simulink model "mdl_pm_foc_allpu_alternative"  (R2024a)
settings: Solver=FixedStepAuto  StartTime=0.0  StopTime=1  FixedStep=1e-5  RelTol=1e-3
undefined symbols (not defined in the file): param, sigbuilder_block
libraries: spsControlledVoltageSourceLib x3, spsPermanentMagnetSynchronousMachineLib x1, spsGroundLib x1, sps_lib x1
settings Model: Creator=jack  LastModifiedBy=steve
settings SolverCC: ZeroCrossControl=DisableAll  ZeroCrossAlgorithm=Adaptive
settings OptimizationCC: ReuseModelBlockBuffer=off
settings DebuggingCC: MaskedZcDiagnostic=none  IgnoredZcDiagnostic=none
settings RTWCC: GPUComputeCapability=3.5

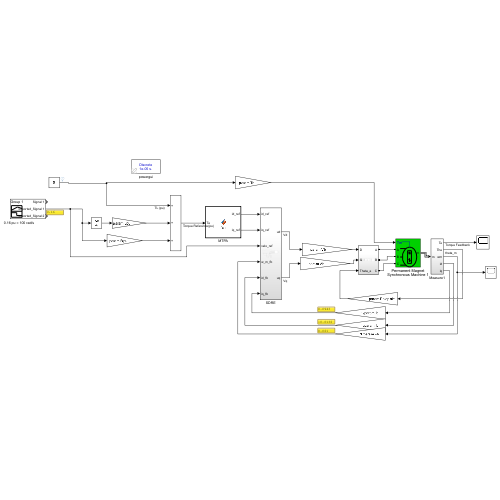
[thumbnail: Simulink's stored preview of the top-level diagram]
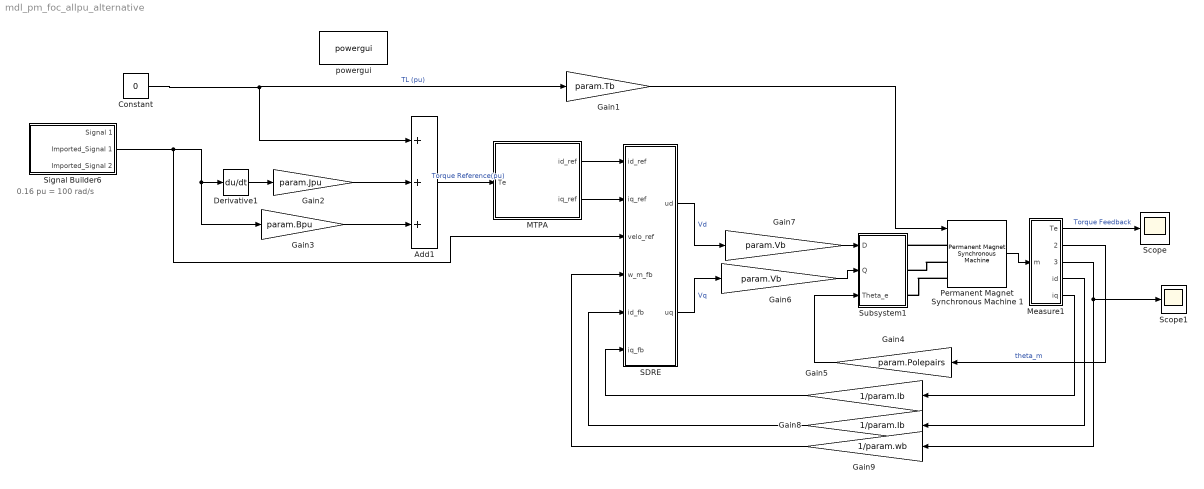
== system mdl_pm_foc_allpu_alternative ==
  note: 0.16 pu = 100 rad/s
  Add1 : Sum  Inputs=+++
  Constant : Constant  Value=0
  Derivative1 : Derivative
  Gain1 : Gain  Gain=param.Tb
  Gain2 : Gain  Gain=param.Jpu
  Gain3 : Gain  Gain=param.Bpu
  Gain4 : Gain  Gain=param.Polepairs
  Gain5 : Gain  Gain=1/param.Ib
  Gain6 : Gain  Gain=param.Vb
  Gain7 : Gain  Gain=param.Vb
  Gain8 : Gain  Gain=1/param.Ib
  Gain9 : Gain  Gain=1/param.wb
  MTPA : MATLAB Function  TreatAsAtomicUnit=on
  Measure1 : Subsystem
  Permanent Magnet Synchronous Machine 1 : spsPermanentMagnetSynchronousMachineLib/Permanent Magnet Synchronous Machine  NbPhases=3  FluxDistribution=Sinusoidal  RotorType=Salient-pole  MechanicalLoad=Torque Tm  PresetModel=No  ShowDetailedParameters=on  MeasurementBus=off  Resistance=param.Rs  Inductance=8.5e-3  dqInductances=[param.Ld param.Lq]  La=5.7e-3  MachineConstant=Flux linkage established by magnets (V.s)  Flux=param.Lamda_f  VoltageCst=164.1942  TorqueCst=1.3579  Flat=120  Mechanical=[param.J param.B param.Polepairs]  PolePairs=4  InitialConditions=[0,0, 0,0]  InitialConditions5ph=[0 0 0 0 0 0]  RefAngle=Aligned with phase A axis (original Park)  IterativeDiscreteModel=Trapezoidal non iterative  TsBlock=param.timestep  TsPowergui=0
  SDRE : Subsystem
  Scope : Scope
  Scope1 : Scope
  Signal Builder6 : Subsystem  Tag=STV Subsys  LoadFcn=sigbuilder_block('load');  StartFcn=sigbuilder_block('start');  StopFcn=sigbuilder_block('stop');  ClipboardFcn=sigbuilder_block('clipboard');  mask(Sigbuilder block){tuvar=[0:10]}
      mask help: Simulink:masks:SigbuilderBlock_MD
      mask init:
      | if ~strcmp(get_param(bdroot(gcbh),'SimulationStatus'),'stopped') tuvar = sigbuilder_block('maskInit'); end
      settings: CopyFcn=sigbuilder_block('copy');  DeleteFcn=sigbuilder_block('delete');  ModelCloseFcn=sigbuilder_block('modelClose');  PreSaveFcn=sigbuilder_block('preSave');  PauseFcn=sigbuilder_block('pause');  ContinueFcn=sigbuilder_block('continue');  NameChangeFcn=sigbuilder_block('namechange');  OpenFcn=sigbuilder_block('open',[6 0 1428 711.75 ]);  CloseFcn=sigbuilder_block('close');
      mask Display: plot(0, 0, 100, 100,[2, 2, 32, 32, 2], [68, 8, 8, 68, 68],[32, 2], [38, 38], [32, 19, 2],[53, 60, 44], [32, 17, 17, 2],[16, 16, 31, 31]);txt = getActiveGroup(gcbh);text(2, 100, txt,'verticalAlignment', 'top');
  Subsystem1 : Subsystem
  powergui : sps_lib/powergui  Priority=1  SimulationMode=Discrete  SampleTime=1e-05  frequency=60  Iterations=50  frequencyindice=0  Pbase=100e6  ErrMax=1e-4  UnitsV=kV  UnitsW=MW  buscounter=0  FunctionMessages=off  echomessages=off  EnableUseOfTLC=off  CurrentSourceSwitches=off  DisableSnubberDevices=off  DisableRonSwitches=off  DisableVfSwitches=off  DisplayEquations=off  AutomaticDiscreteSolvers=off  SolverType=Tustin/Backward Euler (TBE)  Interpol=off  ExternalGateDelay=off  methode=off  Ts=100  x0status=blocks  SPID=on  SwTol=0  HookPort=off  NonlinearTolerance=1e-4  nMaxIteration=100  ContinueOnMaxIteration=off  RestoreLinks=warning  ResistiveCurrentMeasurement=off  Frange=[0:2:500]  Ylog=off  Xlog=on  ShowGrid=off  save=off  variable=ZData  structure=0  ZoomFFT=off  StartTime=0.0  cycles=1  DisplayStyle=1  fundamental=60  FreqAxis=off  MaxFrequency=1000  frequencyindicesteady=1  RmsSteady=1  display=off
  wires:
  Constant/1 -> Add1/1, Gain1/1  "TL (pu)"
  Gain3/1 -> Add1/3
  Add1/1 -> MTPA/1(Te)  "Torque Reference(pu)"
  Gain2/1 -> Add1/2
  Signal Builder6/2(Imported_Signal 1) -> Gain3/1, Derivative1/1, SDRE/3(velo_ref)
  MTPA/1(id_ref) -> SDRE/1(id_ref)
  Derivative1/1 -> Gain2/1
  MTPA/2(iq_ref) -> SDRE/2(iq_ref)
  SDRE/2(uq) -> Gain6/1  "Vq"
  SDRE/1(ud) -> Gain7/1  "Vd"
  Permanent Magnet Synchronous Machine 1/1 -> Measure1/1(m)
  Gain1/1 -> Permanent Magnet Synchronous Machine 1/1
  Measure1/2(The) -> Gain4/1  "theta_m"
  Gain4/1 -> Subsystem1/3(Theta_e)
  Gain6/1 -> Subsystem1/2(Q)
  Gain7/1 -> Subsystem1/1(D)
  Measure1/5(iq) -> Gain5/1
  Measure1/4(id) -> Gain8/1
  Gain5/1 -> SDRE/6(iq_fb)
  Gain8/1 -> SDRE/5(id_fb)
  Gain9/1 -> SDRE/4(w_m_fb)
  Measure1/1(Te) -> Scope/1  "Torque Feedback"
  Measure1/3(wm) -> Scope1/1, Gain9/1
  connections:
  Permanent Magnet Synchronous Machine 1/LConn3 -- Subsystem1/RConn3
  Permanent Magnet Synchronous Machine 1/LConn2 -- Subsystem1/RConn2
  Permanent Magnet Synchronous Machine 1/LConn1 -- Subsystem1/RConn1

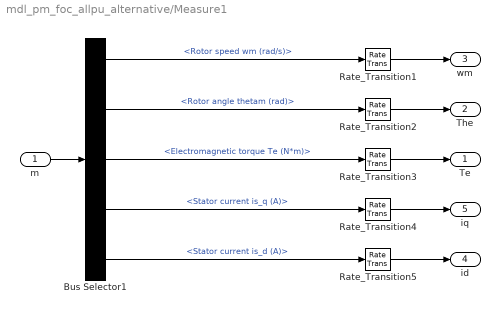
== system mdl_pm_foc_allpu_alternative/Measure1 ==
  m : Inport
  Bus Selector1 : BusSelector  OutputSignals=Rotor speed wm (rad/s),Rotor angle thetam (rad),Electromagnetic torque Te (N*m),Stator current is_q (A),Stator current is_d (A)
  Rate_Transition{1..5} (5 alike) : RateTransition  Integrity=off
  Te : Outport
  The : Outport  Port=2
  wm : Outport  Port=3
  id : Outport  Port=4
  iq : Outport  Port=5
  wires:
  Bus Selector1/1 -> Rate_Transition1/1  "<Rotor speed wm (rad/s)>"
  m/1 -> Bus Selector1/1
  Bus Selector1/3 -> Rate_Transition3/1  "<Electromagnetic torque Te (N*m)>"
  Bus Selector1/2 -> Rate_Transition2/1  "<Rotor angle thetam (rad)>"
  Rate_Transition1/1 -> wm/1
  Rate_Transition2/1 -> The/1
  Rate_Transition3/1 -> Te/1
  Bus Selector1/4 -> Rate_Transition4/1  "<Stator current is_q (A)>"
  Rate_Transition4/1 -> iq/1
  Bus Selector1/5 -> Rate_Transition5/1  "<Stator current is_d (A)>"
  Rate_Transition5/1 -> id/1

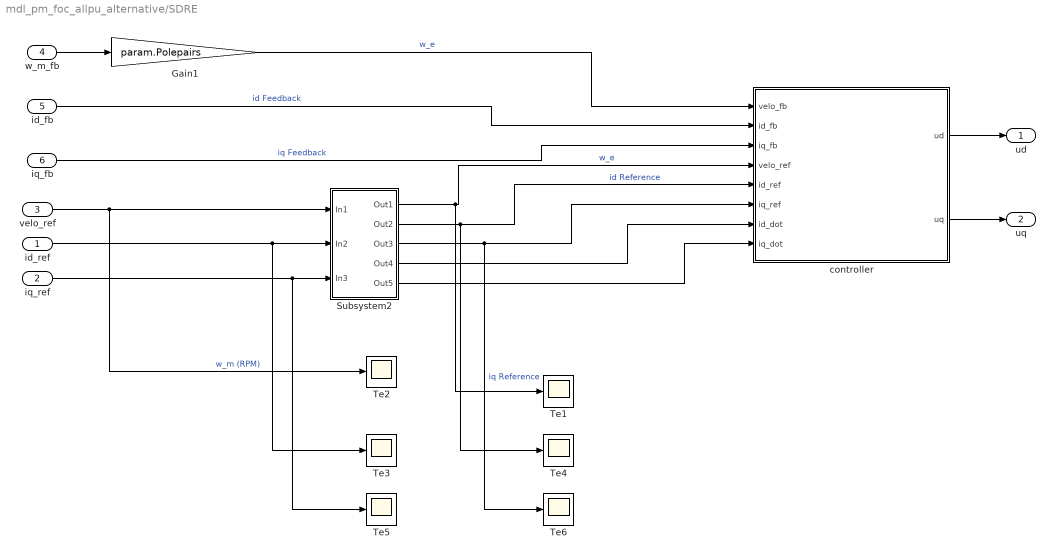
== system mdl_pm_foc_allpu_alternative/SDRE ==
  id_ref : Inport
  iq_ref : Inport  Port=2
  velo_ref : Inport  Port=3
  w_m_fb : Inport  Port=4
  id_fb : Inport  Port=5
  iq_fb : Inport  Port=6
  Gain1 : Gain  Gain=param.Polepairs
  Subsystem2 : Subsystem
  Te{1..6} (6 alike) : Scope
  controller : MATLAB Function  TreatAsAtomicUnit=on
  ud : Outport
  uq : Outport  Port=2
  wires:
  controller/2(uq) -> uq/1
  controller/1(ud) -> ud/1
  iq_ref/1 -> Te5/1, Subsystem2/3(In3)
  id_ref/1 -> Te3/1, Subsystem2/2(In2)
  velo_ref/1 -> Te2/1, Subsystem2/1(In1)  "w_m (RPM)"
  Subsystem2/5(Out5) -> controller/8(iq_dot)
  Subsystem2/4(Out4) -> controller/7(id_dot)
  Subsystem2/1(Out1) -> Te1/1, controller/4(velo_ref)  "w_e"
  Subsystem2/2(Out2) -> controller/5(id_ref), Te4/1  "id Reference"
  Subsystem2/3(Out3) -> Te6/1, controller/6(iq_ref)  "iq Reference"
  id_fb/1 -> controller/2(id_fb)  "id Feedback"
  iq_fb/1 -> controller/3(iq_fb)  "iq Feedback"
  Gain1/1 -> controller/1(velo_fb)  "w_e"
  w_m_fb/1 -> Gain1/1

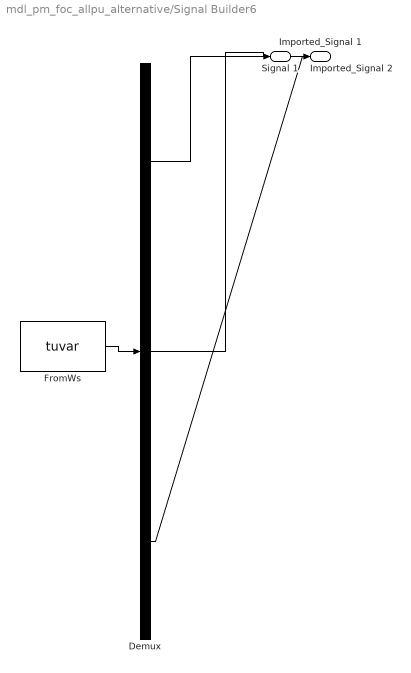
== system mdl_pm_foc_allpu_alternative/Signal Builder6 ==
  Demux : Demux  Tag=STV Demux  Outputs=3
      settings: DisplayOption=none
  FromWs : FromWorkspace  Tag=STV FromWs  VariableName=tuvar
      SigBuilderData=|
      | common.afterFinalStr = 'Extrapolate'
      | common.sampleTime = 0
      | dataSet.timeRange = [0 1]
      | dataSet.name = 'Group 1'
      | sbobj.Groups.Name = 'Group 1'
      | sbobj.Groups.Signals(1).Name = 'Signal 1'
      | sbobj.Groups.Signals(1).XData = [0 1]
      | sbobj.Groups.Signals(1).YData = [0 0]
      | sbobj.Groups.Signals(2).Name = 'Imported_Signal 1'
      | sbobj.Groups.Signals(2).XData = [0 0.005 0.4 0.46 0.52 0.58 0.8 1]
      | sbobj.Groups.Signals(2).YData = [0 0.159 0.16 0.16 0.16 0.16 0.16 0.16]
      | sbobj.Groups.Signals(3).Name = 'Imported_Signal 2'
      | sbobj.Groups.Signals(3).XData = [0 0.2 0.4 0.46 0.72 0.78 0.9 1]
      | sbobj.Groups.Signals(3).YData = [0 -900 -900 850 900 -900 -900 0]
      | sbobj.Groups.TimeRange = [0 1]
  Signal 1 : Outport  Tag=STV Outport
  Imported_Signal 1 : Outport  Tag=STV Outport  Port=2
  Imported_Signal 2 : Outport  Tag=STV Outport  Port=3
  wires:
  FromWs/1 -> Demux/1
  Demux/1 -> Signal 1/1
  Demux/2 -> Imported_Signal 1/1
  Demux/3 -> Imported_Signal 2/1

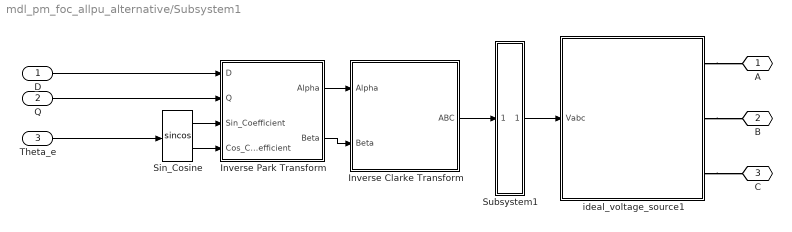
== system mdl_pm_foc_allpu_alternative/Subsystem1 ==
  D : Inport
  Q : Inport  Port=2
  Theta_e : Inport  Port=3
  Inverse Clarke Transform : Subsystem
  Inverse Park Transform : Subsystem
  Sin_Cosine : Trigonometry  Operator=sincos
  Subsystem1 : Subsystem
      mask Display: fprintf('D/C')
  ideal_voltage_source1 : Subsystem  VariantControl=variantPwm == enumPwm.behavior
  A : PMIOPort  Side=Right
  B : PMIOPort  Port=2  Side=Right
  C : PMIOPort  Port=3  Side=Right
  wires:
  D/1 -> Inverse Park Transform/1(D)
  Inverse Park Transform/1(Alpha) -> Inverse Clarke Transform/1(Alpha)
  Sin_Cosine/1 -> Inverse Park Transform/3(Sin_Coefficient)
  Theta_e/1 -> Sin_Cosine/1
  Sin_Cosine/2 -> Inverse Park Transform/4(Cos_Coefficient)
  Inverse Park Transform/2(Beta) -> Inverse Clarke Transform/2(Beta)
  Subsystem1/1(Out1) -> ideal_voltage_source1/1(Vabc)
  Inverse Clarke Transform/1(ABC) -> Subsystem1/1(In1)
  Q/1 -> Inverse Park Transform/2(Q)
  connections:
  ideal_voltage_source1/RConn2 -- B/RConn1
  ideal_voltage_source1/RConn3 -- C/RConn1
  ideal_voltage_source1/RConn1 -- A/RConn1

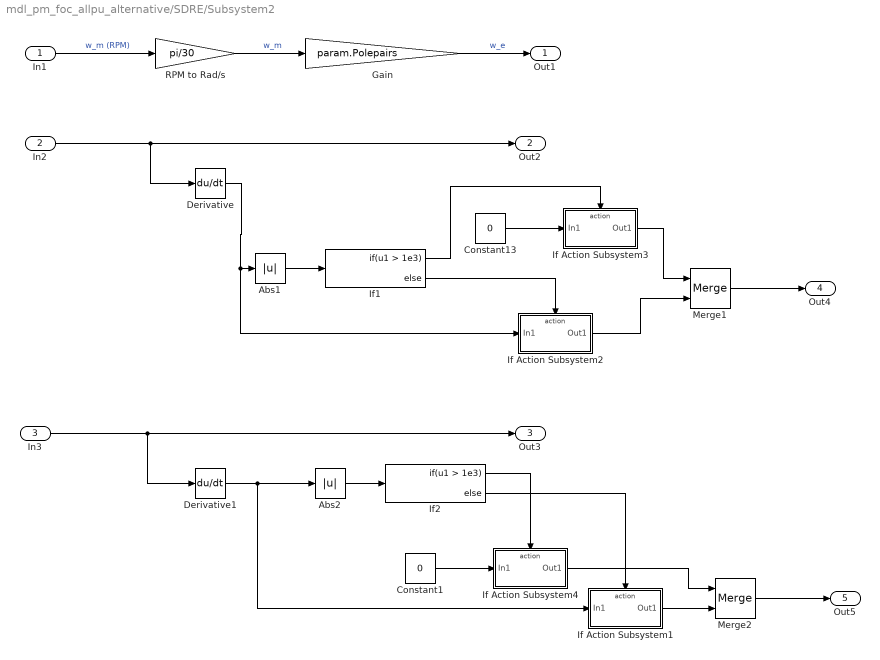
== system mdl_pm_foc_allpu_alternative/SDRE/Subsystem2 ==
  In1 : Inport
  In2 : Inport  Port=2
  In3 : Inport  Port=3
  Abs1 : Abs  SaturateOnIntegerOverflow=off
  Abs2 : Abs  SaturateOnIntegerOverflow=off
  Constant1 : Constant  Value=0
  Constant13 : Constant  Value=0
  Derivative : Derivative
  Derivative1 : Derivative
  Gain : Gain  Gain=param.Polepairs
  If Action Subsystem1 : Subsystem  TreatAsAtomicUnit=on
  If Action Subsystem2 : Subsystem  TreatAsAtomicUnit=on
  If Action Subsystem3 : Subsystem  TreatAsAtomicUnit=on
  If Action Subsystem4 : Subsystem  TreatAsAtomicUnit=on
  If1 : If  IfExpression=u1 > 1e3
  If2 : If  IfExpression=u1 > 1e3
  Merge1 : Merge
  Merge2 : Merge
  RPM to Rad/s : Gain  Gain=pi/30
  Out1 : Outport
  Out2 : Outport  Port=2
  Out3 : Outport  Port=3
  Out4 : Outport  Port=4
  Out5 : Outport  Port=5
  wires:
  Derivative1/1 -> If Action Subsystem1/1(In1), Abs2/1
  In3/1 -> Out3/1, Derivative1/1
  In1/1 -> RPM to Rad/s/1  "w_m (RPM)"
  In2/1 -> Out2/1, Derivative/1
  If Action Subsystem2/1(Out1) -> Merge1/2
  If1/1 -> If Action Subsystem3/Action
  Abs1/1 -> If1/1
  Constant13/1 -> If Action Subsystem3/1(In1)
  Derivative/1 -> If Action Subsystem2/1(In1), Abs1/1
  If1/2 -> If Action Subsystem2/Action
  If Action Subsystem3/1(Out1) -> Merge1/1
  Merge1/1 -> Out4/1
  Constant1/1 -> If Action Subsystem4/1(In1)
  If2/2 -> If Action Subsystem1/Action
  Merge2/1 -> Out5/1
  If2/1 -> If Action Subsystem4/Action
  If Action Subsystem4/1(Out1) -> Merge2/1
  If Action Subsystem1/1(Out1) -> Merge2/2
  Abs2/1 -> If2/1
  RPM to Rad/s/1 -> Gain/1  "w_m"
  Gain/1 -> Out1/1  "w_e"

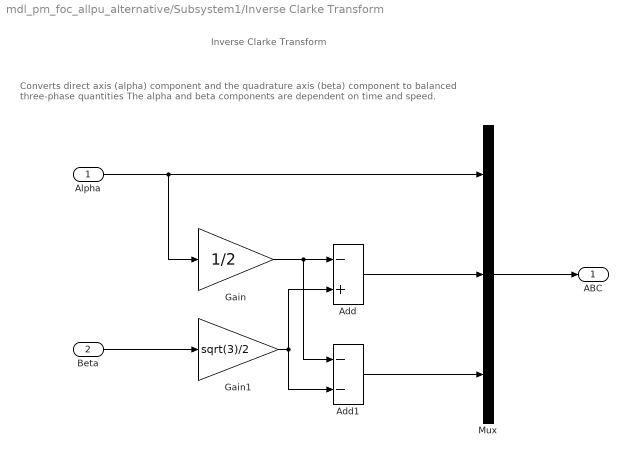
== system mdl_pm_foc_allpu_alternative/Subsystem1/Inverse Clarke Transform ==
  note: Inverse Clarke Transform
  note: Converts direct axis (alpha) component and the quadrature axis (beta) component to balanced three-phase quantities
      | The alpha and beta components are dependent on time and speed.
  Alpha : Inport
  Beta : Inport  Port=2
  Add : Sum  Inputs=-+  OutDataTypeStr=Inherit: Same as first input
  Add1 : Sum  Inputs=--  OutDataTypeStr=Inherit: Same as first input
  Gain : Gain  Gain=1/2
  Gain1 : Gain  Gain=sqrt(3)/2
  Mux : Mux  Inputs=3
  ABC : Outport  VectorParamsAs1DForOutWhenUnconnected=off
  wires:
  Beta/1 -> Gain1/1
  Mux/1 -> ABC/1
  Alpha/1 -> Mux/1, Gain/1
  Add1/1 -> Mux/3
  Gain1/1 -> Add1/2, Add/2
  Gain/1 -> Add1/1, Add/1
  Add/1 -> Mux/2

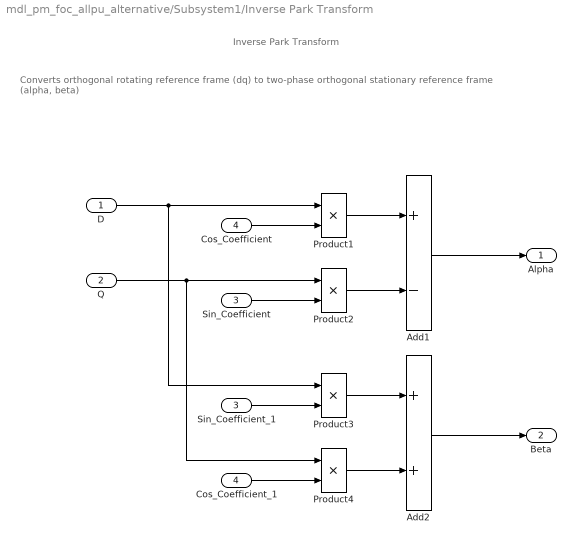
== system mdl_pm_foc_allpu_alternative/Subsystem1/Inverse Park Transform ==
  note: Converts orthogonal rotating reference frame (dq) to two-phase orthogonal stationary reference frame (alpha, beta)
  note: Inverse Park Transform
  D : Inport
  Q : Inport  Port=2
  Sin_Coefficient : Inport  Port=3
  Cos_Coefficient : Inport  Port=4
  Add1 : Sum  Inputs=+-  OutDataTypeStr=Inherit: Same as first input
  Add2 : Sum  OutDataTypeStr=Inherit: Same as first input
  Cos_Coefficient_1 : InportShadow  Port=4
  Product{1..4} (4 alike) : Product  RndMeth=Simplest
  Sin_Coefficient_1 : InportShadow  Port=3
  Alpha : Outport  VectorParamsAs1DForOutWhenUnconnected=off
  Beta : Outport  Port=2  VectorParamsAs1DForOutWhenUnconnected=off
  wires:
  Sin_Coefficient_1/1 -> Product3/2
  Product2/1 -> Add1/2
  Cos_Coefficient_1/1 -> Product4/2
  Add2/1 -> Beta/1
  Product3/1 -> Add2/1
  Add1/1 -> Alpha/1
  Product1/1 -> Add1/1
  Product4/1 -> Add2/2
  Sin_Coefficient/1 -> Product2/2
  D/1 -> Product3/1, Product1/1
  Q/1 -> Product2/1, Product4/1
  Cos_Coefficient/1 -> Product1/2

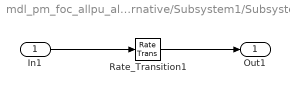
== system mdl_pm_foc_allpu_alternative/Subsystem1/Subsystem1 ==
  In1 : Inport
  Rate_Transition1 : RateTransition  Integrity=off
  Out1 : Outport  VectorParamsAs1DForOutWhenUnconnected=off
  wires:
  In1/1 -> Rate_Transition1/1
  Rate_Transition1/1 -> Out1/1

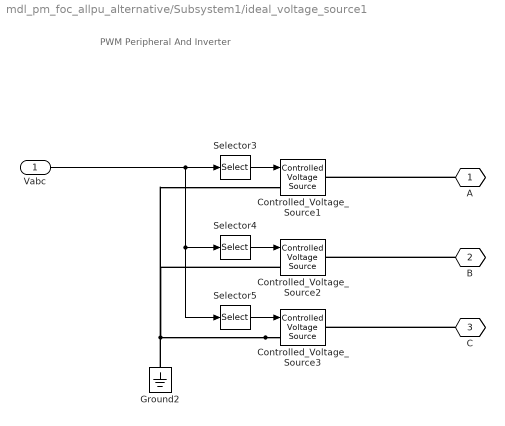
== system mdl_pm_foc_allpu_alternative/Subsystem1/ideal_voltage_source1 ==
  note: PWM Peripheral And Inverter
  Vabc : Inport
  Controlled_Voltage_Source1 : spsControlledVoltageSourceLib/Controlled Voltage Source  Initialize=off  Source_Type=DC  Amplitude=12  Phase=0  Frequency=0  Measurements=None
  Controlled_Voltage_Source2 : spsControlledVoltageSourceLib/Controlled Voltage Source  Initialize=off  Source_Type=DC  Amplitude=12  Phase=0  Frequency=0  Measurements=None
  Controlled_Voltage_Source3 : spsControlledVoltageSourceLib/Controlled Voltage Source  Initialize=off  Source_Type=DC  Amplitude=12  Phase=0  Frequency=0  Measurements=None
  Ground2 : spsGroundLib/Ground  LConnTagsString=a
  Selector3 : Selector  InputPortWidth=3  IndexOptions=Index vector (dialog)  Indices=[1]  OutputSizes=1
  Selector4 : Selector  InputPortWidth=3  IndexOptions=Index vector (dialog)  Indices=2  OutputSizes=1
  Selector5 : Selector  InputPortWidth=3  IndexOptions=Index vector (dialog)  Indices=3  OutputSizes=1
  A : PMIOPort  Tag=PMCPort  Side=Right
  B : PMIOPort  Tag=PMCPort  Port=2  Side=Right
  C : PMIOPort  Tag=PMCPort  Port=3  Side=Right
  wires:
  Vabc/1 -> Selector4/1, Selector5/1, Selector3/1
  Selector5/1 -> Controlled_Voltage_Source3/1
  Selector4/1 -> Controlled_Voltage_Source2/1
  Selector3/1 -> Controlled_Voltage_Source1/1
  connections:
  C/RConn1 -- Controlled_Voltage_Source3/RConn1
  B/RConn1 -- Controlled_Voltage_Source2/RConn1
  A/RConn1 -- Controlled_Voltage_Source1/RConn1
  Controlled_Voltage_Source3/LConn1 -- Controlled_Voltage_Source1/LConn1 -- Controlled_Voltage_Source2/LConn1 -- Ground2/LConn1

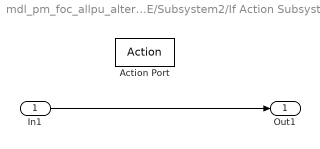
== system mdl_pm_foc_allpu_alternative/SDRE/Subsystem2/If Action Subsystem1 ==
  In1 : Inport
  Action Port : ActionPort  ActionPortLabel=else
  Out1 : Outport
  wires:
  In1/1 -> Out1/1

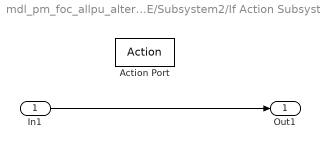
== system mdl_pm_foc_allpu_alternative/SDRE/Subsystem2/If Action Subsystem2 ==
  In1 : Inport
  Action Port : ActionPort  ActionPortLabel=else
  Out1 : Outport
  wires:
  In1/1 -> Out1/1

== system mdl_pm_foc_allpu_alternative/SDRE/Subsystem2/If Action Subsystem3 ==
  In1 : Inport
  Action Port : ActionPort  ActionPortLabel=if(u1 > 1e3)
  Out1 : Outport
  wires:
  In1/1 -> Out1/1

== system mdl_pm_foc_allpu_alternative/SDRE/Subsystem2/If Action Subsystem4 ==
  In1 : Inport
  Action Port : ActionPort  ActionPortLabel=if(u1 > 1e3)
  Out1 : Outport
  wires:
  In1/1 -> Out1/1

== matlab function mdl_pm_foc_allpu_alternative/SDRE/controller ==
  settings: updateMethod=DISCRETE
  data: velo_fb input; id_fb input; iq_fb input; velo_ref input; id_ref input; iq_ref input; ud output; uq output; id_dot input; iq_dot input; param parameter
function [ud, uq] = SDRE_motor(velo_fb, id_fb, iq_fb, velo_ref, id_ref, iq_ref, id_dot, iq_dot, param)

% 獲取電機參數
timestep    = param.timestep;
Ld          = param.Ld;
Lq          = param.Lq;
Rs          = param.Rs;
Lamda_m     = param.Lamda_f;
pole        = param.pole;
Ib          = param.Ib;
Vb          = param.Vb;
wb          = param.wb;
Rspu        = param.Rspu;
Xdpu        = param.Xdpu;
Xqpu        = param.Xqpu;
Lamda_fpu   = param.Lamda_fpu;
Jpu         = param.Jpu;
Bpu         = param.Bpu;


persistent z_state
persistent Ts
%-------------------------------------------------------------------------------

% 初始化 z 狀態為 1
if isempty(z_state)
    z_state = 1;
end

% 自動取得取樣週期（僅限模擬模式有效）
if isempty(Ts)
    Ts = timestep;
end

% 更新 z 狀態
eta = 10;  % 衰減係數，可根據設計調整
z_state = z_state + Ts * (-eta * z_state);

%-------------------------------------------------------------------------------


if isempty(id_dot)
    id_dot = 0;
    iq_dot = 0;
end

velo_error = velo_fb - velo_ref;
id_error = id_fb - id_ref;
iq_error = iq_fb - iq_ref;

if isempty(iq_error)
    velo_error = 0;
    id_error = 0;
    iq_error = 0;
end

%-------------------------------------------------------------------------------
% 組成誤差向量（含 z 狀態）
error = [velo_error iq_error id_error z_state];

k1 = (pole*Lamda_fpu)/(2*Jpu);
k2 = Bpu/Jpu;
k3 = pole/(2*Jpu);
k4 = (wb*Rspu)/Xqpu;
k5 = (wb*Lamda_fpu)/Xqpu;
k6 = wb/Xqpu;
k7 = (wb*Rspu)/Xdpu;
k8 = wb/Xdpu;
k9 = (wb*Xqpu)/Xdpu;
k10 = (wb*Xdpu)/Xqpu;
k11 = (2*(Xdpu-Xqpu))/(2*Jpu);
% 狀態矩陣 A
A11 = -k2; 
A12 = k1; 
A13 = k11*iq_fb;

A21 = -k5-k10*id_fb; 
A22 = -k4; 
A23 = 0;

A31 = k9*iq_fb; 
A32 = 0; 
A33 = -k7;

A14 =  (1/z_state)*k11*iq_error*id_ref;
A24 = -(1/z_state)*k10*id_error*velo_ref;
A34 =  (1/z_state)*k9*iq_error*velo_ref;
A44 = - eta;

A41 = 0;
A42 = 0;
A43 = 0;

A = [A11 A12 A13 A14;
     A21 A22 A23 A24;
     A31 A32 A33 A34;
     A41 A42 A43 A44];

% 控制矩陣 B
B = [0    0;
     k6   0;
     0   k8;
     0    0];


% Q, R 矩陣
rate = sqrt(iq_error^2 + id_error^2);
Q = diag([5000, 1 + exp(-rate), 10000 + exp(-rate), 100]);  % z 的權重 100，可調
R = diag([1 1]);

%-------------------------------------------------------------------------------

% 解 SDRE 控制律
[P_ss_care, ~] = SDA_CARE(A, B, Q, R);
u_redeem = -inv(R) * B' * P_ss_care * error';

% 計算基礎電壓
ucq = (Ib*Rs/Vb) * iq_ref + (wb*Lamda_m)* velo_ref + (Ib*Lq) * iq_dot + (Ld*Ib*wb) * id_error * velo_ref + (Ld*Ib*wb) * velo_fb * id_ref;
ucd = (Ib*Rs) * id_ref + (Ib*Ld) * id_dot - (Ib*wb*Lq) * iq_error * velo_ref - (Lq*Ib*wb) * velo_fb * iq_ref;

if ucq > 1e5
    ucq = 0;
end
if ucd > 1e5
    ucd = 0;
end

% 最終控制電壓
uq = ucq + u_redeem(1);
ud = ucd + u_redeem(2);

% 保證輸出型態
ud = reshape(ud, 1, 1);
uq = reshape(uq, 1, 1);

end

== matlab function mdl_pm_foc_allpu_alternative/MTPA ==
  data: id_ref output; Te input; iq_ref output; param parameter
function [id_ref , iq_ref] = fcn(Te, param)

% 獲取電機參數
Ld          = param.Ld;
Lq          = param.Lq;
Lamda_m     = param.Lamda_f;
pole        = param.pole;
Ib          = param.Ib;
Tb          = param.Tb;

Ldq = Ld-Lq;

%Lambda_m = Lambda_m *pi/30;
p1 = 3*pole*Ldq^2 /(4*Lamda_m);
p2 = 0;
p3 = (3*pole*Lamda_m)/(4*Ib);
p4 = -(Tb/(Ib)^3)*Te;
p = [p1 p2 p3 p4];
r = roots(p);

real_solutions = r(imag(r) == 0);


iq_ref = real(max(real_solutions));
id_ref = Ib*Ldq*(iq_ref^2) /Lamda_m;
end
